simulink model "prj"  (R2020b)
settings: Solver=VariableStepAuto  StartTime=0.0  StopTime=100.0  RelTol=1e-3
values from neighbouring files (symbols this model uses):
  C0 = 0.008    [data.m]
  C1 = 1.6e-6    (= 1.6e-06)    [data.m]
  Cx = 1.2    [data.m]
  D = 3    [data.m]
  g = 9.81    [data.m]
  m = 3    [data.m]
  rho = 1.225    [data.m]
  S = 0.0739    [data.m]
libraries: simulink x2, powerlib_meascontrol x1
settings Model: Creator=xoxox  LastModifiedBy=xoxox

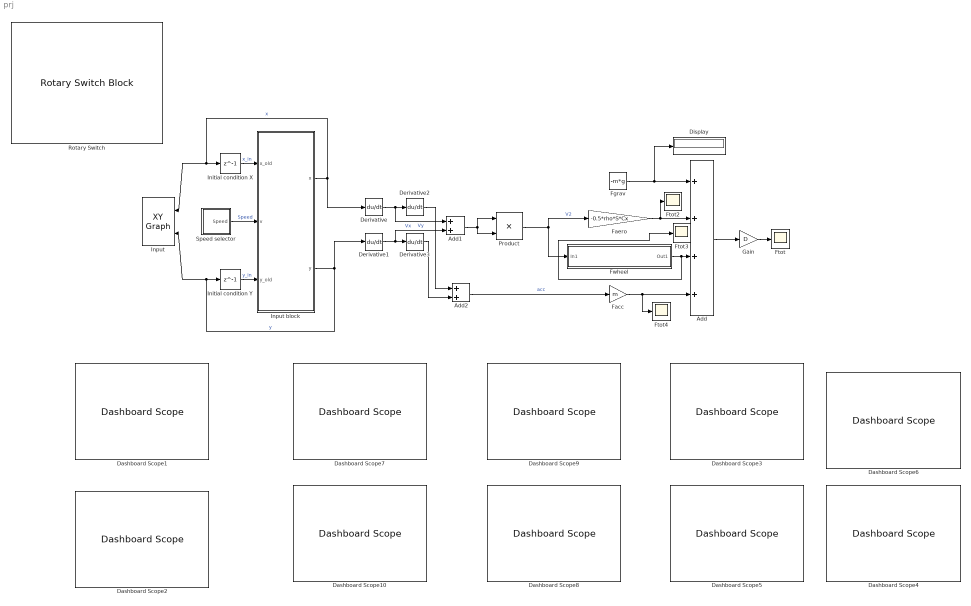
== system prj ==
  Add : Sum  Inputs=++++
  Add1 : Sum
  Add2 : Sum
  Dashboard Scope{1..10} (10 alike) : DashboardScope
  Derivative{,1..3} (4 alike) : Derivative
  Display : Display
  Facc : Gain  Gain=m
  Faero : Gain  Gain=-0.5*rho*S*Cx
  Fgrav : Constant  Value=-m*g
  Ftot{,2..4} (4 alike) : Scope
  Fwheel : Subsystem
  Gain : Gain  Gain=D
  Initial condition X : Delay  DelayLength=1
  Initial condition Y : Delay  DelayLength=1
  Input : simulink/Sinks/XY Graph  xmin=-1  xmax=5.5  ymin=-5  ymax=20  st=-1
  Input block : MATLAB Function  TreatAsAtomicUnit=on
  Product : Product
  Rotary Switch : RotarySwitchBlock
      settings: Values={{'Constant', 'Sine', 'Pulse', 'Ramp', 'Triangle'}, [1 2 3 4 5]}
  Speed selector : Subsystem
  wires:
  Derivative/1 -> Add1/1, Derivative2/1  "Vy"
  Derivative1/1 -> Add1/2, Derivative3/1  "Vx"
  Add/1 -> Gain/1
  Faero/1 -> Ftot2/1, Add/2
  Product/1 -> Faero/1, Fwheel/1(In1)  "V2"
  Fwheel/1(Out1) -> Ftot3/1, Add/3
  Facc/1 -> Ftot4/1, Add/4
  Add1/1 -> Product/2, Product/1
  Derivative2/1 -> Add2/1
  Derivative3/1 -> Add2/2
  Add2/1 -> Facc/1  "acc"
  Input block/2(y) -> Input/2, Initial condition Y/1, Derivative1/1  "y"
  Speed selector/1(Speed) -> Input block/2(v)  "Speed"
  Input block/1(x) -> Derivative/1, Initial condition X/1, Input/1  "x"
  Initial condition X/1 -> Input block/1(x_old)  "x_in"
  Initial condition Y/1 -> Input block/3(y_old)  "y_in"
  Gain/1 -> Ftot/1
  Fgrav/1 -> Display/1, Add/1

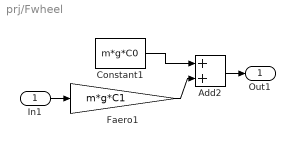
== system prj/Fwheel ==
  In1 : Inport
  Add2 : Sum
  Constant1 : Constant  Value=m*g*C0
  Faero1 : Gain  Gain=m*g*C1
  Out1 : Outport
  wires:
  Faero1/1 -> Add2/2
  Add2/1 -> Out1/1
  Constant1/1 -> Add2/1
  In1/1 -> Faero1/1

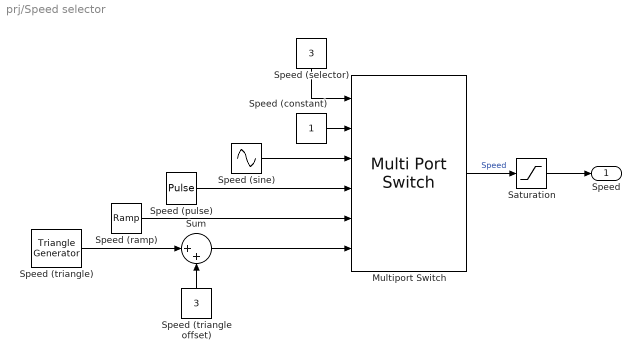
== system prj/Speed selector ==
  Multiport Switch : MultiPortSwitch  Inputs=5
  Saturation : Saturate  UpperLimit=4.664899955035971
  Speed (constant) : Constant
  Speed (pulse) : DiscretePulseGenerator  PulseType=Time based  Period=10  PulseWidth=50
  Speed (ramp) : simulink/Sources/Ramp  slope=1  start=0  InitialOutput=0
  Speed (selector) : Constant  Value=3
  Speed (sine) : Sin  Bias=1  SampleTime=0
  Speed (triangle offset) : Constant  Value=3
  Speed (triangle) : powerlib_meascontrol/Pulse & Signal Generators/Triangle Generator  Freq=1/30  Phase=90  Ts=0
  Sum : Sum  Inputs=|++
  Speed : Outport
  wires:
  Speed (triangle offset)/1 -> Sum/2
  Sum/1 -> Multiport Switch/6
  Speed (pulse)/1 -> Multiport Switch/4
  Speed (triangle)/1 -> Sum/1
  Speed (sine)/1 -> Multiport Switch/3
  Speed (constant)/1 -> Multiport Switch/2
  Speed (selector)/1 -> Multiport Switch/1
  Speed (ramp)/1 -> Multiport Switch/5
  Multiport Switch/1 -> Saturation/1  "Speed"
  Saturation/1 -> Speed/1

== matlab function prj/Input block ==
  data: x output; x_old input; v input; y_old input; y output
function [x, y] = input(x_old , v , y_old)

    h = 10; %Straight line distance
    d = 5; %"Circle" diameter
    
    Ts = 0.01; %MUST also Simulink sample time

    is_on_part_1_flag = ((x_old == 0 && y_old < h));
    is_on_part_2_flag = ((x_old < d && y_old >= h));
    is_on_part_3_flag = ((x_old >= d && y_old >=0));
    is_on_part_4_flag = (~is_on_part_1_flag &&...
                         ~is_on_part_2_flag &&...
                         ~is_on_part_3_flag);
  
                     
         
    x = is_on_part_1_flag * (0)+...
        is_on_part_2_flag * (x_old + Ts*v)+... 
        is_on_part_3_flag * (d)+...
        is_on_part_4_flag * ((x_old - Ts*v > 0)*(x_old - Ts*v)); %Ternary operator workaround

    y = is_on_part_1_flag * (y_old + Ts*v)+...
        is_on_part_2_flag * (h + (d/2)*sin(pi*x/d))+... 
        is_on_part_3_flag * (y_old - Ts*v)+...
        is_on_part_4_flag * (- (d/2)*sin(pi*x/d));    

         
%     x = is_on_part_1_flag * (0)+...
%         is_on_part_2_flag * (timestamp*v)+... 
%         is_on_part_3_flag * (d)+...
%         is_on_part_4_flag * ((d - timestamp*v >0)*(d - timestamp*v));
%    
%     y = is_on_part_1_flag * (timestamp*v)+...
%         is_on_part_2_flag * (h + (d/2) * sin(pi*timestamp*v/d))+... 
%         is_on_part_3_flag * (h-timestamp*v)+...
%         is_on_part_4_flag * (-(d/2) * sin(pi*timestamp*v/d));
 

            
            


end
